simulink model "syntheses"  (R2015b)
settings: Solver=FixedStepDiscrete  SolverMode=SingleTasking  StartTime=0.0  StopTime=sim_len  FixedStep=1  RelTol=1e-3
values from neighbouring files (symbols this model uses):
  N_sub = 16    [synthese_params.m]
undefined symbols (not defined in the file or in its folder): modulator_reg_1_address, modulator_reg_1_default, modulator_reg_1_num_bits
undefined symbols (not defined in the file): reset_reg_address
libraries: xbsIndex_r4 x136
settings Model: Creator=randy  LastModifiedBy=randy

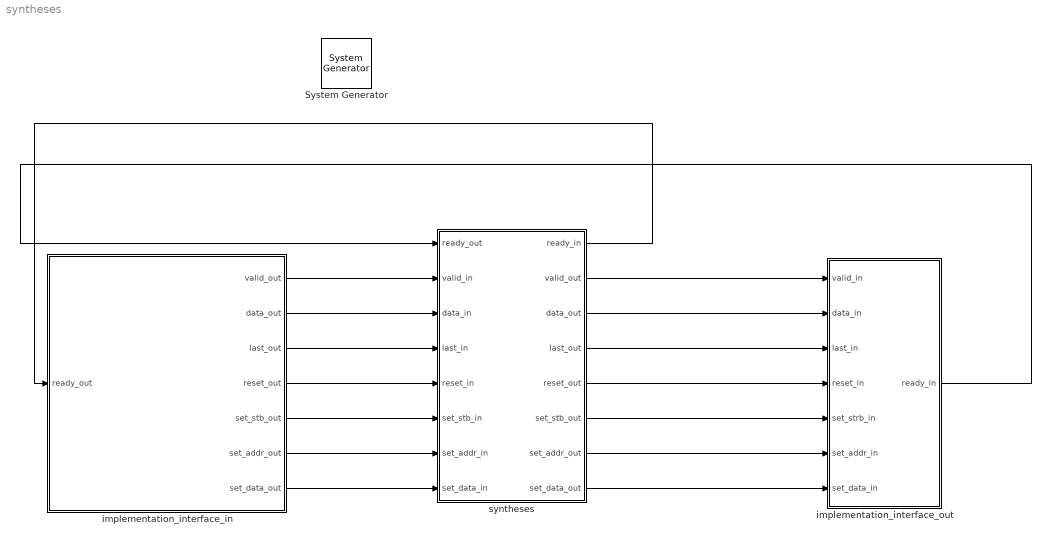
== system syntheses ==
  " System Generator" : xbsIndex_r4/ System Generator  Tag=genX  xilinxfamily=kintex7  part=xc7k410t  speed=-2  package=ffg900  synthesis_tool=Vivado  clock_wrapper=Clock Enables  directory=./checkpoint  proj_type=Vivado  Synth_file=Vivado Synthesis Defaults  Impl_file=Vivado Implementation Defaults  testbench=off  simulink_period=1  sysclk_period=5  dcm_input_clock_period=10  incr_netlist=off  trim_vbits=Everywhere in SubSystem  dbl_ovrd=According to Block Masks  core_generation=According to Block Masks  run_coregen=off  deprecated_control=off  eval_field=0  block_type=sysgen
  implementation_interface_in : Subsystem
  implementation_interface_out : Subsystem
  syntheses : Subsystem
  wires:
  implementation_interface_in/1(valid_out) -> syntheses/2(valid_in)
  implementation_interface_in/2(data_out) -> syntheses/3(data_in)
  implementation_interface_in/3(last_out) -> syntheses/4(last_in)
  syntheses/1(ready_in) -> implementation_interface_in/1(ready_out)
  syntheses/2(valid_out) -> implementation_interface_out/1(valid_in)
  syntheses/3(data_out) -> implementation_interface_out/2(data_in)
  syntheses/4(last_out) -> implementation_interface_out/3(last_in)
  implementation_interface_out/1(ready_in) -> syntheses/1(ready_out)
  implementation_interface_in/4(reset_out) -> syntheses/5(reset_in)
  implementation_interface_in/5(set_stb_out) -> syntheses/6(set_stb_in)
  implementation_interface_in/6(set_addr_out) -> syntheses/7(set_addr_in)
  implementation_interface_in/7(set_data_out) -> syntheses/8(set_data_in)
  syntheses/5(reset_out) -> implementation_interface_out/4(reset_in)
  syntheses/6(set_stb_out) -> implementation_interface_out/5(set_strb_in)
  syntheses/7(set_addr_out) -> implementation_interface_out/6(set_addr_in)
  syntheses/8(set_data_out) -> implementation_interface_out/7(set_data_in)

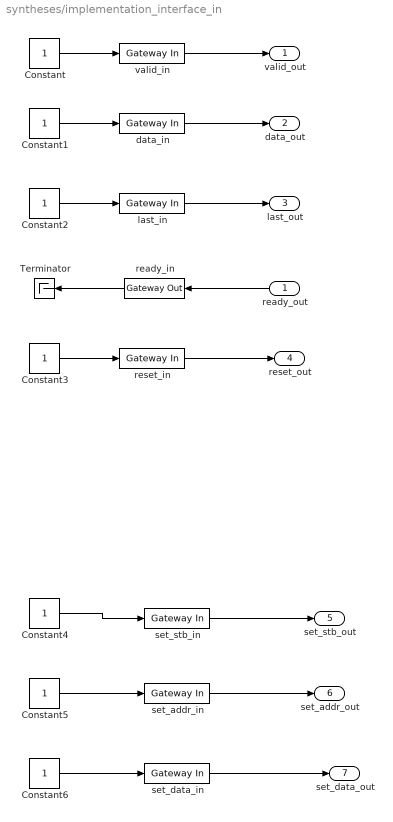
== system syntheses/implementation_interface_in ==
  ready_out : Inport
  Constant{,1..6} (7 alike) : Constant
  Terminator : Terminator
  data_in : xbsIndex_r4/Gateway In  gui_display_data_type=Fixed-point  arith_type=Unsigned  n_bits=32  bin_pt=0  preci_type=Single  exp_width=8  frac_width=24  rows=1  columns=1  quantization="Round  (unbiased: +/- Inf)"  overflow=Saturate  period=1  UseAsADC=off  ADCChannel='1'  interface=None  automatic_assignment=on  address_offset=hex2dec('00')  intf_name=''  intf_description=''  timing_constraint=None  locs_specified=off  LOCs={}  io_standard={}  inherit_from_input=off  hdl_port=on  dbl_ovrd=off  block_type=gatewayin
  last_in : xbsIndex_r4/Gateway In  gui_display_data_type=Boolean  arith_type=Boolean  n_bits=16  bin_pt=14  preci_type=Single  exp_width=8  frac_width=24  rows=1  columns=1  quantization="Round  (unbiased: +/- Inf)"  overflow=Saturate  period=1  UseAsADC=off  ADCChannel='1'  interface=None  automatic_assignment=on  address_offset=hex2dec('00')  intf_name=''  intf_description=''  timing_constraint=None  locs_specified=off  LOCs={}  io_standard={}  inherit_from_input=off  hdl_port=on  dbl_ovrd=off  block_type=gatewayin
  ready_in : xbsIndex_r4/Gateway Out  inherit_from_input=off  hdl_port=on  rows=1  columns=1  UseAsDAC=off  DACChannel='1'  interface=None  automatic_assignment=on  address_offset=hex2dec('00')  intf_name=''  intf_description=''  timing_constraint=None  locs_specified=off  LOCs={}  io_standard={}  block_type=gatewayout
  reset_in : xbsIndex_r4/Gateway In  gui_display_data_type=Boolean  arith_type=Boolean  n_bits=16  bin_pt=14  preci_type=Single  exp_width=8  frac_width=24  rows=1  columns=1  quantization="Round  (unbiased: +/- Inf)"  overflow=Saturate  period=1  UseAsADC=off  ADCChannel='1'  interface=None  automatic_assignment=on  address_offset=hex2dec('00')  intf_name=''  intf_description=''  timing_constraint=None  locs_specified=off  LOCs={}  io_standard={}  inherit_from_input=off  hdl_port=on  dbl_ovrd=off  block_type=gatewayin
  set_addr_in : xbsIndex_r4/Gateway In  gui_display_data_type=Fixed-point  arith_type=Unsigned  n_bits=8  bin_pt=0  preci_type=Single  exp_width=8  frac_width=24  rows=1  columns=1  quantization="Round  (unbiased: +/- Inf)"  overflow=Saturate  period=1  UseAsADC=off  ADCChannel='1'  interface=None  automatic_assignment=on  address_offset=hex2dec('00')  intf_name=''  intf_description=''  timing_constraint=None  locs_specified=off  LOCs={}  io_standard={}  inherit_from_input=off  hdl_port=on  dbl_ovrd=off  block_type=gatewayin
  set_data_in : xbsIndex_r4/Gateway In  gui_display_data_type=Fixed-point  arith_type=Unsigned  n_bits=32  bin_pt=0  preci_type=Single  exp_width=8  frac_width=24  rows=1  columns=1  quantization="Round  (unbiased: +/- Inf)"  overflow=Saturate  period=1  UseAsADC=off  ADCChannel='1'  interface=None  automatic_assignment=on  address_offset=hex2dec('00')  intf_name=''  intf_description=''  timing_constraint=None  locs_specified=off  LOCs={}  io_standard={}  inherit_from_input=off  hdl_port=on  dbl_ovrd=off  block_type=gatewayin
  set_stb_in : xbsIndex_r4/Gateway In  gui_display_data_type=Boolean  arith_type=Boolean  n_bits=16  bin_pt=14  preci_type=Single  exp_width=8  frac_width=24  rows=1  columns=1  quantization="Round  (unbiased: +/- Inf)"  overflow=Saturate  period=1  UseAsADC=off  ADCChannel='1'  interface=None  automatic_assignment=on  address_offset=hex2dec('00')  intf_name=''  intf_description=''  timing_constraint=None  locs_specified=off  LOCs={}  io_standard={}  inherit_from_input=off  hdl_port=on  dbl_ovrd=off  block_type=gatewayin
  valid_in : xbsIndex_r4/Gateway In  gui_display_data_type=Boolean  arith_type=Boolean  n_bits=16  bin_pt=14  preci_type=Single  exp_width=8  frac_width=24  rows=1  columns=1  quantization="Round  (unbiased: +/- Inf)"  overflow=Saturate  period=1  UseAsADC=off  ADCChannel='1'  interface=None  automatic_assignment=on  address_offset=hex2dec('00')  intf_name=''  intf_description=''  timing_constraint=None  locs_specified=off  LOCs={}  io_standard={}  inherit_from_input=off  hdl_port=on  dbl_ovrd=off  block_type=gatewayin
  valid_out : Outport
  data_out : Outport  Port=2
  last_out : Outport  Port=3
  reset_out : Outport  Port=4
  set_stb_out : Outport  Port=5
  set_addr_out : Outport  Port=6
  set_data_out : Outport  Port=7
  wires:
  set_stb_in/1 -> set_stb_out/1
  set_addr_in/1 -> set_addr_out/1
  set_data_in/1 -> set_data_out/1
  reset_in/1 -> reset_out/1
  ready_out/1 -> ready_in/1
  last_in/1 -> last_out/1
  data_in/1 -> data_out/1
  valid_in/1 -> valid_out/1
  ready_in/1 -> Terminator/1
  Constant/1 -> valid_in/1
  Constant1/1 -> data_in/1
  Constant3/1 -> reset_in/1
  Constant2/1 -> last_in/1
  Constant4/1 -> set_stb_in/1
  Constant5/1 -> set_addr_in/1
  Constant6/1 -> set_data_in/1

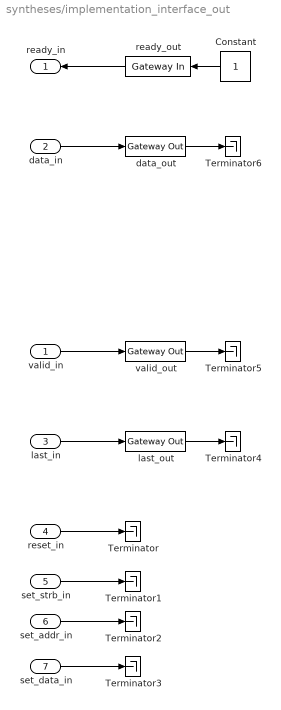
== system syntheses/implementation_interface_out ==
  valid_in : Inport
  data_in : Inport  Port=2
  last_in : Inport  Port=3
  reset_in : Inport  Port=4
  set_strb_in : Inport  Port=5
  set_addr_in : Inport  Port=6
  set_data_in : Inport  Port=7
  Constant : Constant
  Terminator{,1..6} (7 alike) : Terminator
  data_out : xbsIndex_r4/Gateway Out  inherit_from_input=off  hdl_port=on  rows=1  columns=1  UseAsDAC=off  DACChannel='1'  interface=None  automatic_assignment=on  address_offset=hex2dec('00')  intf_name=''  intf_description=''  timing_constraint=None  locs_specified=off  LOCs={}  io_standard={}  block_type=gatewayout
  last_out : xbsIndex_r4/Gateway Out  inherit_from_input=off  hdl_port=on  rows=1  columns=1  UseAsDAC=off  DACChannel='1'  interface=None  automatic_assignment=on  address_offset=hex2dec('00')  intf_name=''  intf_description=''  timing_constraint=None  locs_specified=off  LOCs={}  io_standard={}  block_type=gatewayout
  ready_out : xbsIndex_r4/Gateway In  gui_display_data_type=Boolean  arith_type=Boolean  n_bits=16  bin_pt=14  preci_type=Single  exp_width=8  frac_width=24  rows=1  columns=1  quantization="Round  (unbiased: +/- Inf)"  overflow=Saturate  period=1  UseAsADC=off  ADCChannel='1'  interface=None  automatic_assignment=on  address_offset=hex2dec('00')  intf_name=''  intf_description=''  timing_constraint=None  locs_specified=off  LOCs={}  io_standard={}  inherit_from_input=off  hdl_port=on  dbl_ovrd=off  block_type=gatewayin
  valid_out : xbsIndex_r4/Gateway Out  inherit_from_input=off  hdl_port=on  rows=1  columns=1  UseAsDAC=off  DACChannel='1'  interface=None  automatic_assignment=on  address_offset=hex2dec('00')  intf_name=''  intf_description=''  timing_constraint=None  locs_specified=off  LOCs={}  io_standard={}  block_type=gatewayout
  ready_in : Outport
  wires:
  valid_out/1 -> Terminator5/1
  Constant/1 -> ready_out/1
  last_out/1 -> Terminator4/1
  data_out/1 -> Terminator6/1
  reset_in/1 -> Terminator/1
  set_strb_in/1 -> Terminator1/1
  set_addr_in/1 -> Terminator2/1
  set_data_in/1 -> Terminator3/1
  valid_in/1 -> valid_out/1
  data_in/1 -> data_out/1
  last_in/1 -> last_out/1
  ready_out/1 -> ready_in/1

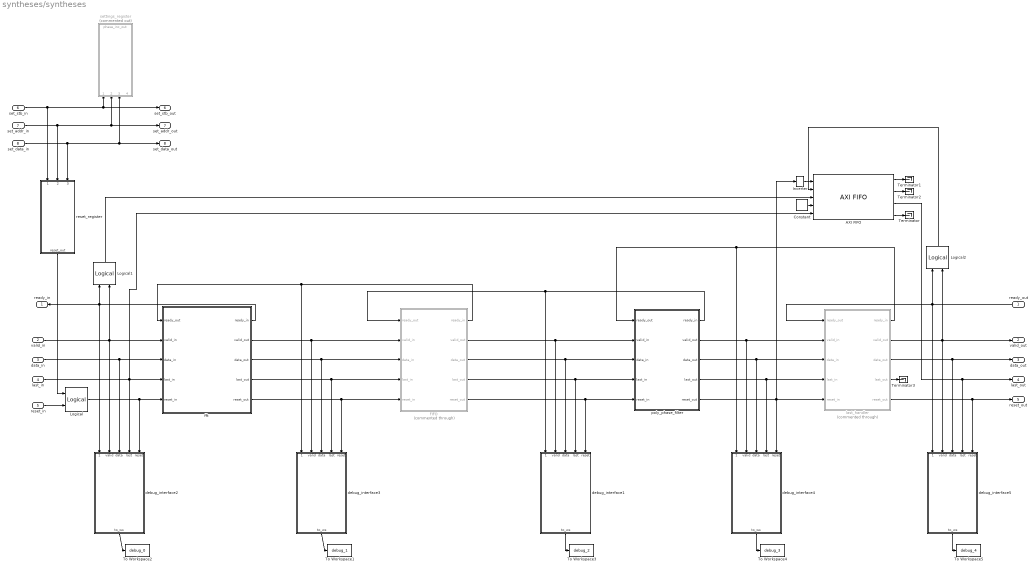
== system syntheses/syntheses ==
  ready_out : Inport
  valid_in : Inport  Port=2
  data_in : Inport  Port=3
  last_in : Inport  Port=4
  reset_in : Inport  Port=5
  set_stb_in : Inport  Port=6
  set_addr_in : Inport  Port=7
  set_data_in : Inport  Port=8
  AXI FIFO : xbsIndex_r4/AXI FIFO  input_depth_axis=4K  actual_fifo_depth_label=4098  enable_tdata=on  enable_tdest=off  enable_tstrb=off  enable_tready=on  enable_tid=off  enable_tuser=off  enable_tkeep=off  enable_tlast=on  has_aresetn=on  enable_data_counts_axis=off  fifo_implementation_type_axis=Common Clock Block RAM  trim_axipin_name=on  programmable_full_type_axis=Full  full_threshold_assert_value_axis=0  programmable_empty_type_axis=Empty  empty_threshold_assert_value_axis=1022  underflow_flag_axi=0  underflow_sense_axi=Active High  overflow_flag_axi=0  overflow_sense_axi=Active High  block_type=axi_fifo
  Constant : xbsIndex_r4/Constant  const=1.0  gui_display_data_type=Fixed-point  arith_type=Unsigned  n_bits=8  bin_pt=0  preci_type=Single  exp_width=8  frac_width=24  explicit_period=on  period=1  equ=P=C  opselect=C  inp2=PCIN>>17  opr=+  inp1=P  carry=CIN  dbl_ovrd=off  block_type=constant
  FIFO : Subsystem  Commented=through
  Inverter : xbsIndex_r4/Inverter  en=off  latency=0  dbl_ovrd=off  block_type=inv
  Logical : xbsIndex_r4/Logical  logical_function=OR  inputs=2  en=off  latency=0  precision=Full  arith_type=Unsigned  n_bits=16  bin_pt=0  align_bp=on  dbl_ovrd=off  block_type=logical
  Logical1 : xbsIndex_r4/Logical  logical_function=AND  inputs=2  en=off  latency=0  precision=Full  arith_type=Unsigned  n_bits=16  bin_pt=0  align_bp=on  dbl_ovrd=off  block_type=logical
  Logical2 : xbsIndex_r4/Logical  logical_function=AND  inputs=2  en=off  latency=0  precision=Full  arith_type=Unsigned  n_bits=16  bin_pt=0  align_bp=on  dbl_ovrd=off  block_type=logical
  Terminator{,1..3} (4 alike) : Terminator
  To Workspace1 : ToWorkspace  VariableName=debug_1  SaveFormat=Timeseries  SampleTime=-1
  To Workspace2 : ToWorkspace  VariableName=debug_0  SaveFormat=Timeseries  SampleTime=-1
  To Workspace3 : ToWorkspace  VariableName=debug_2  SaveFormat=Timeseries  SampleTime=-1
  To Workspace4 : ToWorkspace  VariableName=debug_3  SaveFormat=Timeseries  SampleTime=-1
  To Workspace5 : ToWorkspace  VariableName=debug_4  SaveFormat=Timeseries  SampleTime=-1
  debug_interface1 : Subsystem
  debug_interface2 : Subsystem
  debug_interface3 : Subsystem
  debug_interface4 : Subsystem
  debug_interface5 : Subsystem
  fft : Subsystem
  last_handler : Subsystem  Commented=through
  poly_phase_filter : Subsystem
  reset_register : Subsystem  mask{address=reset_reg_address}
  settings_register : Subsystem  Commented=on
  ready_in : Outport
  valid_out : Outport  Port=2
  data_out : Outport  Port=3
  last_out : Outport  Port=4
  reset_out : Outport  Port=5
  set_stb_out : Outport  Port=6
  set_addr_out : Outport  Port=7
  set_data_out : Outport  Port=8
  wires:
  set_addr_in/1 -> settings_register/2(set_addr), set_addr_out/1, reset_register/2(set_addr)
  set_data_in/1 -> settings_register/3(set_data), set_data_out/1, reset_register/3(set_data)
  debug_interface2/1(to_ws) -> To Workspace2/1
  debug_interface3/1(to_ws) -> To Workspace1/1
  debug_interface1/1(to_ws) -> To Workspace3/1
  debug_interface4/1(to_ws) -> To Workspace4/1
  fft/1(ready_in) -> Logical1/1, debug_interface2/1(ready), ready_in/1
  data_in/1 -> debug_interface2/3(data), fft/3(data_in)
  valid_in/1 -> Logical1/2, debug_interface2/2(valid), fft/2(valid_in)
  fft/2(valid_out) -> debug_interface3/2(valid), FIFO/2(valid_in)
  fft/3(data_out) -> debug_interface3/3(data), FIFO/3(data_in)
  fft/4(last_out) -> debug_interface3/4(last), FIFO/4(last_in)
  fft/5(reset_out) -> debug_interface3/5(reset), FIFO/5(reset_in)
  FIFO/2(valid_out) -> debug_interface1/2(valid), poly_phase_filter/2(valid_in)
  FIFO/3(data_out) -> debug_interface1/3(data), poly_phase_filter/3(data_in)
  FIFO/4(last_out) -> debug_interface1/4(last), poly_phase_filter/4(last_in)
  FIFO/5(reset_out) -> debug_interface1/5(reset), poly_phase_filter/5(reset_in)
  poly_phase_filter/1(ready_in) -> debug_interface1/1(ready), FIFO/1(ready_out)
  FIFO/1(ready_in) -> debug_interface3/1(ready), fft/1(ready_out)
  debug_interface5/1(to_ws) -> To Workspace5/1
  poly_phase_filter/2(valid_out) -> debug_interface4/2(valid), last_handler/2(valid_in)
  poly_phase_filter/3(data_out) -> last_handler/3(data_in), debug_interface4/3(data)
  poly_phase_filter/4(last_out) -> debug_interface4/4(last), last_handler/4(last_in)
  poly_phase_filter/5(reset_out) -> debug_interface4/5(reset), last_handler/5(reset_in), Inverter/1
  last_handler/1(ready_in) -> poly_phase_filter/1(ready_out), debug_interface4/1(ready)
  ready_out/1 -> Logical2/1, debug_interface5/1(ready), last_handler/1(ready_out)
  last_handler/2(valid_out) -> Logical2/2, debug_interface5/2(valid), valid_out/1
  last_handler/3(data_out) -> data_out/1, debug_interface5/3(data)
  last_handler/5(reset_out) -> reset_out/1, debug_interface5/5(reset)
  Logical/1 -> fft/5(reset_in), debug_interface2/5(reset)
  reset_in/1 -> Logical/2
  reset_register/1(reset_out) -> Logical/1
  set_stb_in/1 -> reset_register/1(set_stb), settings_register/1(set_stb), set_stb_out/1
  last_in/1 -> AXI FIFO/5, fft/4(last_in), debug_interface2/4(last)
  AXI FIFO/1 -> Terminator1/1
  Constant/1 -> AXI FIFO/4
  AXI FIFO/2 -> Terminator2/1
  AXI FIFO/4 -> Terminator/1
  Logical1/1 -> AXI FIFO/3
  Logical2/1 -> AXI FIFO/2
  AXI FIFO/3 -> last_out/1, debug_interface5/4(last)
  last_handler/4(last_out) -> Terminator3/1
  Inverter/1 -> AXI FIFO/1

== system syntheses/syntheses/FIFO ==
  ready_out : Inport
  valid_in : Inport  Port=2
  data_in : Inport  Port=3
  last_in : Inport  Port=4
  reset_in : Inport  Port=5
  AXI FIFO : xbsIndex_r4/AXI FIFO  input_depth_axis=16  actual_fifo_depth_label=18  enable_tdata=on  enable_tdest=off  enable_tstrb=off  enable_tready=on  enable_tid=off  enable_tuser=off  enable_tkeep=off  enable_tlast=on  has_aresetn=on  enable_data_counts_axis=off  fifo_implementation_type_axis=Common Clock Distributed RAM  trim_axipin_name=on  programmable_full_type_axis=Full  full_threshold_assert_value_axis=0  programmable_empty_type_axis=Empty  empty_threshold_assert_value_axis=1022  underflow_flag_axi=0  underflow_sense_axi=Active High  overflow_flag_axi=0  overflow_sense_axi=Active High  block_type=axi_fifo
  Inverter : xbsIndex_r4/Inverter  en=off  latency=0  dbl_ovrd=off  block_type=inv
  ready_in : Outport
  valid_out : Outport  Port=2
  data_out : Outport  Port=3
  last_out : Outport  Port=4
  reset_out : Outport  Port=5
  wires:
  AXI FIFO/1 -> valid_out/1
  data_in/1 -> AXI FIFO/4
  ready_out/1 -> AXI FIFO/2
  last_in/1 -> AXI FIFO/5
  AXI FIFO/3 -> last_out/1
  reset_in/1 -> reset_out/1, Inverter/1
  valid_in/1 -> AXI FIFO/3
  Inverter/1 -> AXI FIFO/1
  AXI FIFO/2 -> data_out/1
  AXI FIFO/4 -> ready_in/1

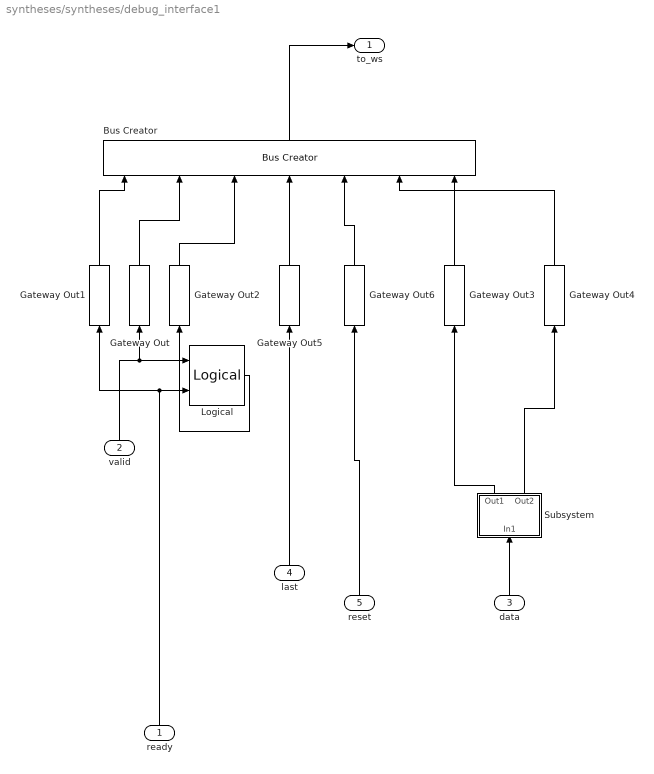
== system syntheses/syntheses/debug_interface1 ==
  ready : Inport
  valid : Inport  Port=2
  data : Inport  Port=3
  last : Inport  Port=4
  reset : Inport  Port=5
  Bus Creator : BusCreator  Inputs=7
  Gateway Out{,1..6} (7 alike) : xbsIndex_r4/Gateway Out  inherit_from_input=off  hdl_port=off  rows=1  columns=1  UseAsDAC=off  DACChannel='1'  interface=None  automatic_assignment=on  address_offset=hex2dec('00')  intf_name=''  intf_description=''  timing_constraint=None  locs_specified=off  LOCs={}  io_standard={}  block_type=gatewayout
  Logical : xbsIndex_r4/Logical  logical_function=AND  inputs=2  en=off  latency=0  precision=Full  arith_type=Unsigned  n_bits=16  bin_pt=0  align_bp=on  dbl_ovrd=off  block_type=logical
  Subsystem : Subsystem
  to_ws : Outport
  wires:
  ready/1 -> Logical/2, Gateway Out1/1
  Gateway Out3/1 -> Bus Creator/7
  Gateway Out2/1 -> Bus Creator/3
  Logical/1 -> Gateway Out2/1
  Gateway Out4/1 -> Bus Creator/6
  valid/1 -> Logical/1, Gateway Out/1
  Gateway Out1/1 -> Bus Creator/1
  Gateway Out/1 -> Bus Creator/2
  Gateway Out6/1 -> Bus Creator/5
  reset/1 -> Gateway Out6/1
  Bus Creator/1 -> to_ws/1
  Subsystem/1(Out1) -> Gateway Out3/1
  Subsystem/2(Out2) -> Gateway Out4/1
  data/1 -> Subsystem/1(In1)
  Gateway Out5/1 -> Bus Creator/4
  last/1 -> Gateway Out5/1

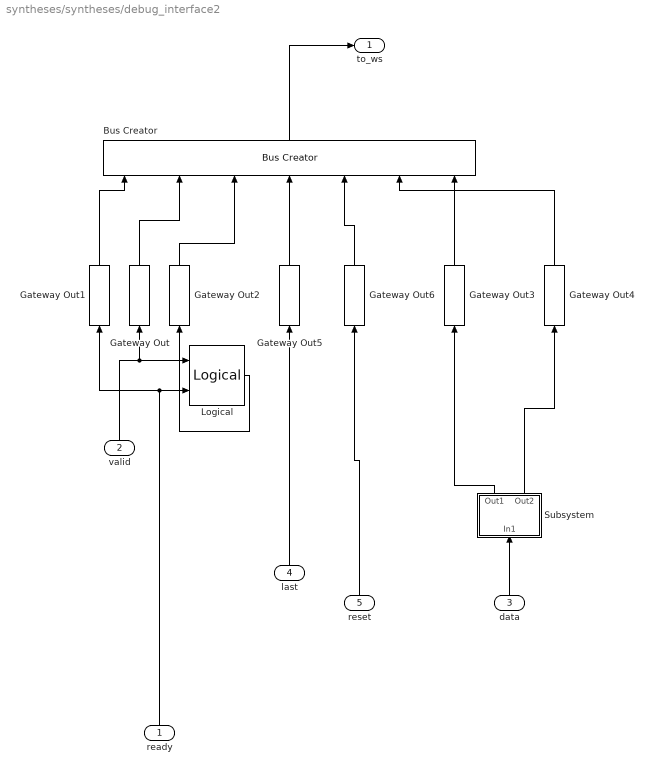
== system syntheses/syntheses/debug_interface2 ==
  ready : Inport
  valid : Inport  Port=2
  data : Inport  Port=3
  last : Inport  Port=4
  reset : Inport  Port=5
  Bus Creator : BusCreator  Inputs=7
  Gateway Out{,1..6} (7 alike) : xbsIndex_r4/Gateway Out  inherit_from_input=off  hdl_port=off  rows=1  columns=1  UseAsDAC=off  DACChannel='1'  interface=None  automatic_assignment=on  address_offset=hex2dec('00')  intf_name=''  intf_description=''  timing_constraint=None  locs_specified=off  LOCs={}  io_standard={}  block_type=gatewayout
  Logical : xbsIndex_r4/Logical  logical_function=AND  inputs=2  en=off  latency=0  precision=Full  arith_type=Unsigned  n_bits=16  bin_pt=0  align_bp=on  dbl_ovrd=off  block_type=logical
  Subsystem : Subsystem
  to_ws : Outport
  wires:
  ready/1 -> Logical/2, Gateway Out1/1
  Gateway Out3/1 -> Bus Creator/7
  Gateway Out2/1 -> Bus Creator/3
  Logical/1 -> Gateway Out2/1
  Gateway Out4/1 -> Bus Creator/6
  valid/1 -> Logical/1, Gateway Out/1
  Gateway Out1/1 -> Bus Creator/1
  Gateway Out/1 -> Bus Creator/2
  Gateway Out6/1 -> Bus Creator/5
  reset/1 -> Gateway Out6/1
  Bus Creator/1 -> to_ws/1
  Subsystem/1(Out1) -> Gateway Out3/1
  Subsystem/2(Out2) -> Gateway Out4/1
  data/1 -> Subsystem/1(In1)
  Gateway Out5/1 -> Bus Creator/4
  last/1 -> Gateway Out5/1

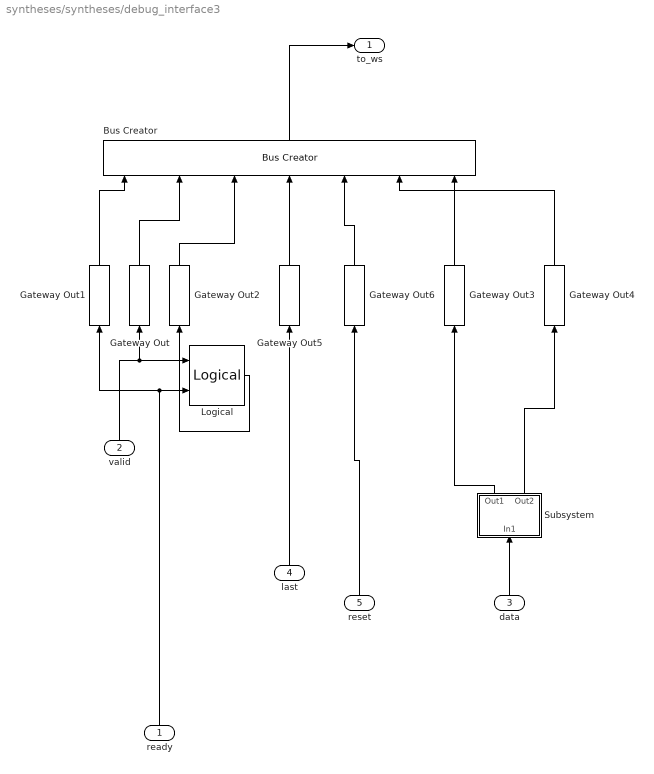
== system syntheses/syntheses/debug_interface3 ==
  ready : Inport
  valid : Inport  Port=2
  data : Inport  Port=3
  last : Inport  Port=4
  reset : Inport  Port=5
  Bus Creator : BusCreator  Inputs=7
  Gateway Out{,1..6} (7 alike) : xbsIndex_r4/Gateway Out  inherit_from_input=off  hdl_port=off  rows=1  columns=1  UseAsDAC=off  DACChannel='1'  interface=None  automatic_assignment=on  address_offset=hex2dec('00')  intf_name=''  intf_description=''  timing_constraint=None  locs_specified=off  LOCs={}  io_standard={}  block_type=gatewayout
  Logical : xbsIndex_r4/Logical  logical_function=AND  inputs=2  en=off  latency=0  precision=Full  arith_type=Unsigned  n_bits=16  bin_pt=0  align_bp=on  dbl_ovrd=off  block_type=logical
  Subsystem : Subsystem
  to_ws : Outport
  wires:
  last/1 -> Gateway Out5/1
  Gateway Out5/1 -> Bus Creator/4
  data/1 -> Subsystem/1(In1)
  Subsystem/2(Out2) -> Gateway Out4/1
  Subsystem/1(Out1) -> Gateway Out3/1
  Bus Creator/1 -> to_ws/1
  reset/1 -> Gateway Out6/1
  Gateway Out6/1 -> Bus Creator/5
  Gateway Out/1 -> Bus Creator/2
  Gateway Out1/1 -> Bus Creator/1
  valid/1 -> Gateway Out/1, Logical/1
  Gateway Out4/1 -> Bus Creator/6
  Logical/1 -> Gateway Out2/1
  Gateway Out2/1 -> Bus Creator/3
  Gateway Out3/1 -> Bus Creator/7
  ready/1 -> Gateway Out1/1, Logical/2

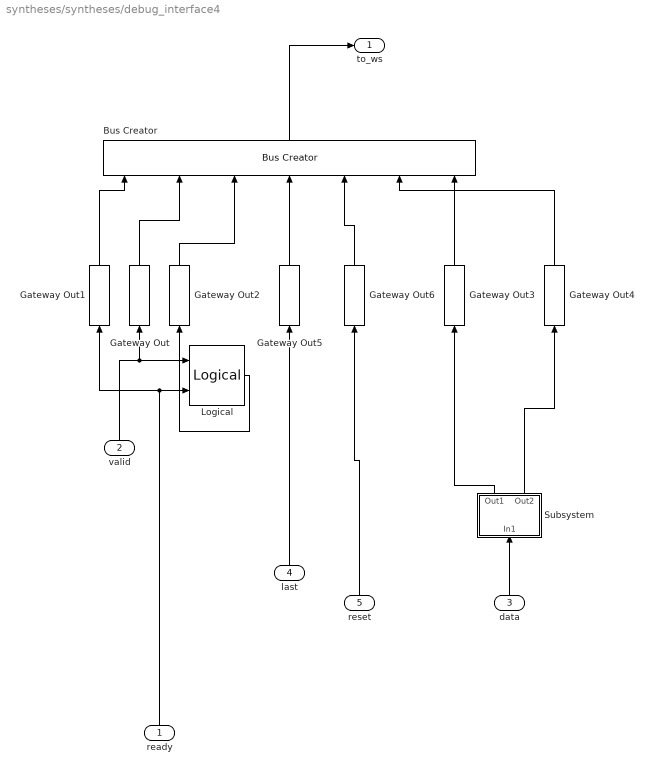
== system syntheses/syntheses/debug_interface4 ==
  ready : Inport
  valid : Inport  Port=2
  data : Inport  Port=3
  last : Inport  Port=4
  reset : Inport  Port=5
  Bus Creator : BusCreator  Inputs=7
  Gateway Out{,1..6} (7 alike) : xbsIndex_r4/Gateway Out  inherit_from_input=off  hdl_port=off  rows=1  columns=1  UseAsDAC=off  DACChannel='1'  interface=None  automatic_assignment=on  address_offset=hex2dec('00')  intf_name=''  intf_description=''  timing_constraint=None  locs_specified=off  LOCs={}  io_standard={}  block_type=gatewayout
  Logical : xbsIndex_r4/Logical  logical_function=AND  inputs=2  en=off  latency=0  precision=Full  arith_type=Unsigned  n_bits=16  bin_pt=0  align_bp=on  dbl_ovrd=off  block_type=logical
  Subsystem : Subsystem
  to_ws : Outport
  wires:
  ready/1 -> Logical/2, Gateway Out1/1
  Gateway Out3/1 -> Bus Creator/7
  Gateway Out2/1 -> Bus Creator/3
  Logical/1 -> Gateway Out2/1
  Gateway Out4/1 -> Bus Creator/6
  valid/1 -> Logical/1, Gateway Out/1
  Gateway Out1/1 -> Bus Creator/1
  Gateway Out/1 -> Bus Creator/2
  Gateway Out6/1 -> Bus Creator/5
  reset/1 -> Gateway Out6/1
  Bus Creator/1 -> to_ws/1
  Subsystem/1(Out1) -> Gateway Out3/1
  Subsystem/2(Out2) -> Gateway Out4/1
  data/1 -> Subsystem/1(In1)
  Gateway Out5/1 -> Bus Creator/4
  last/1 -> Gateway Out5/1

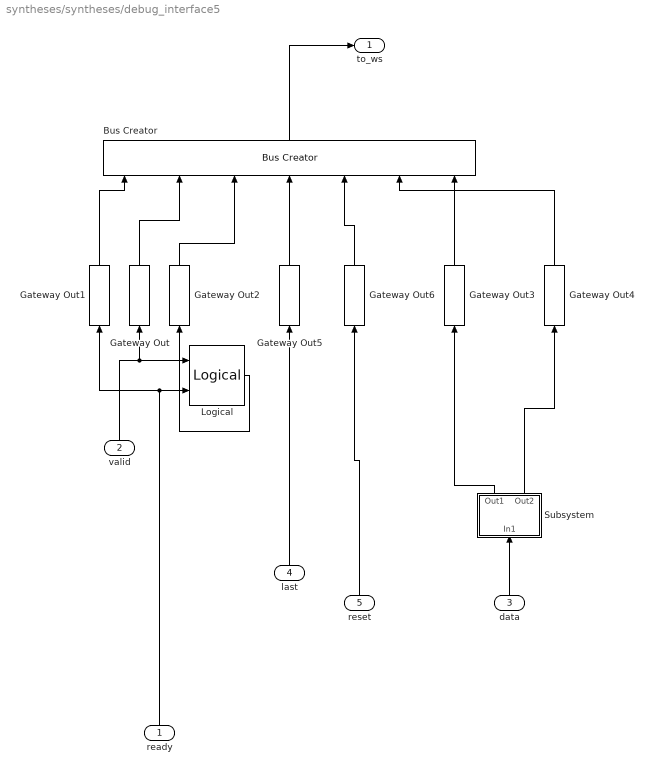
== system syntheses/syntheses/debug_interface5 ==
  ready : Inport
  valid : Inport  Port=2
  data : Inport  Port=3
  last : Inport  Port=4
  reset : Inport  Port=5
  Bus Creator : BusCreator  Inputs=7
  Gateway Out{,1..6} (7 alike) : xbsIndex_r4/Gateway Out  inherit_from_input=off  hdl_port=off  rows=1  columns=1  UseAsDAC=off  DACChannel='1'  interface=None  automatic_assignment=on  address_offset=hex2dec('00')  intf_name=''  intf_description=''  timing_constraint=None  locs_specified=off  LOCs={}  io_standard={}  block_type=gatewayout
  Logical : xbsIndex_r4/Logical  logical_function=AND  inputs=2  en=off  latency=0  precision=Full  arith_type=Unsigned  n_bits=16  bin_pt=0  align_bp=on  dbl_ovrd=off  block_type=logical
  Subsystem : Subsystem
  to_ws : Outport
  wires:
  ready/1 -> Logical/2, Gateway Out1/1
  Gateway Out3/1 -> Bus Creator/7
  Gateway Out2/1 -> Bus Creator/3
  Logical/1 -> Gateway Out2/1
  Gateway Out4/1 -> Bus Creator/6
  valid/1 -> Logical/1, Gateway Out/1
  Gateway Out1/1 -> Bus Creator/1
  Gateway Out/1 -> Bus Creator/2
  Gateway Out6/1 -> Bus Creator/5
  reset/1 -> Gateway Out6/1
  Bus Creator/1 -> to_ws/1
  Subsystem/1(Out1) -> Gateway Out3/1
  Subsystem/2(Out2) -> Gateway Out4/1
  data/1 -> Subsystem/1(In1)
  Gateway Out5/1 -> Bus Creator/4
  last/1 -> Gateway Out5/1

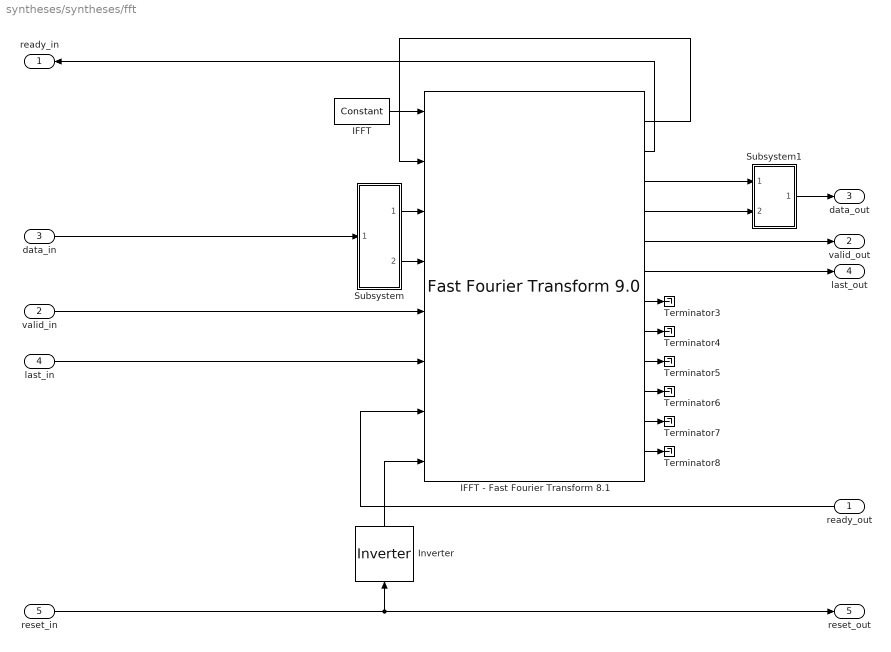
== system syntheses/syntheses/fft ==
  ready_out : Inport
  valid_in : Inport  Port=2
  data_in : Inport  Port=3
  last_in : Inport  Port=4
  reset_in : Inport  Port=5
  IFFT : xbsIndex_r4/Constant  const=0  gui_display_data_type=Fixed-point  arith_type=Unsigned  n_bits=1  bin_pt=0  preci_type=Single  exp_width=8  frac_width=24  explicit_period=off  period=1  equ=P=C  opselect=C  inp2=PCIN>>17  opr=+  inp1=P  carry=CIN  dbl_ovrd=off  block_type=constant
  IFFT - Fast Fourier Transform 8.1 : xbsIndex_r4/Fast Fourier Transform 9.0   transform_length=16  target_clock_frequency=200  target_data_throughput=50  implementation_options=pipelined_streaming_io  run_time_configurable_transform_length=off  phase_factor_width=17  scaling_options=unscaled  rounding_modes=convergent_rounding  aclken=off  aresetn=on  cyclic_prefix_insertion=off  output_ordering=natural_order  throttle_scheme=nonrealtime  xk_index=off  ovflo=off  trim_axipin_name=on  memory_options_data=block_ram  memory_options_phase_factors=block_ram  number_of_stages_using_block_ram_for_data_and_phase_factors=0  memory_options_reorder=block_ram  memory_options_hybrid=off  complex_mult_type=use_mults_resources  butterfly_type=use_xtremedsp_slices  simulation_type=hybrid_sim  simulation_model=sysgen:xfftv9_cmodel  data_path_portlist={ 's_axis_data_tdata', 'm_axis_data_tdata', 'm_axis_status_tdata', 'event_fft_overflow' }  channels=1  input_ordering=natural_order  input_width=16  ip_name=Fast Fourier Transform  ip_version=9.0  dsptool_ready=true  ipcore_usecache=true  ipcore_useipmodelcache=true  wrapper_available=true  port_translation_map={ 'aclken' => 'en', 'aresetn' => 'rst'}  data_format=fixed_point  block_type=xfft_v9_0
  Inverter : xbsIndex_r4/Inverter  en=off  latency=0  dbl_ovrd=off  block_type=inv
  Subsystem : Subsystem
  Subsystem1 : Subsystem
  Terminator{3..8} (6 alike) : Terminator
  ready_in : Outport
  valid_out : Outport  Port=2
  data_out : Outport  Port=3
  last_out : Outport  Port=4
  reset_out : Outport  Port=5
  wires:
  data_in/1 -> Subsystem/1(In1)
  IFFT - Fast Fourier Transform 8.1/10 -> Terminator6/1
  IFFT - Fast Fourier Transform 8.1/11 -> Terminator7/1
  IFFT - Fast Fourier Transform 8.1/8 -> Terminator4/1
  IFFT - Fast Fourier Transform 8.1/9 -> Terminator5/1
  IFFT - Fast Fourier Transform 8.1/7 -> Terminator3/1
  Subsystem/1(imag) -> IFFT - Fast Fourier Transform 8.1/3
  IFFT - Fast Fourier Transform 8.1/12 -> Terminator8/1
  Subsystem/2(real) -> IFFT - Fast Fourier Transform 8.1/4
  IFFT/1 -> IFFT - Fast Fourier Transform 8.1/1
  Subsystem1/1(Out1) -> data_out/1
  IFFT - Fast Fourier Transform 8.1/3 -> Subsystem1/1(imag)
  IFFT - Fast Fourier Transform 8.1/1 -> IFFT - Fast Fourier Transform 8.1/2
  IFFT - Fast Fourier Transform 8.1/4 -> Subsystem1/2(real)
  Inverter/1 -> IFFT - Fast Fourier Transform 8.1/8
  reset_in/1 -> Inverter/1, reset_out/1
  last_in/1 -> IFFT - Fast Fourier Transform 8.1/6
  valid_in/1 -> IFFT - Fast Fourier Transform 8.1/5
  IFFT - Fast Fourier Transform 8.1/2 -> ready_in/1
  IFFT - Fast Fourier Transform 8.1/5 -> valid_out/1
  ready_out/1 -> IFFT - Fast Fourier Transform 8.1/7
  IFFT - Fast Fourier Transform 8.1/6 -> last_out/1

== system syntheses/syntheses/last_handler ==
  ready_out : Inport
  valid_in : Inport  Port=2
  data_in : Inport  Port=3
  last_in : Inport  Port=4
  reset_in : Inport  Port=5
  Constant : xbsIndex_r4/Constant  const=1023  gui_display_data_type=Fixed-point  arith_type=Unsigned  n_bits=nextpow2(1024)  bin_pt=0  preci_type=Single  exp_width=8  frac_width=24  explicit_period=off  period=1  equ=P=C  opselect=C  inp2=PCIN>>17  opr=+  inp1=P  carry=CIN  dbl_ovrd=off  block_type=constant
  Counter : xbsIndex_r4/Counter  cnt_type=Free Running  cnt_to=Inf  operation=Up  start_count=0  cnt_by_val=1  arith_type=Unsigned  n_bits=nextpow2(1024)  bin_pt=0  load_pin=off  rst=on  en=on  explicit_period=on  period=1  use_behavioral_HDL=off  implementation=Fabric  dbl_ovrd=off  block_type=counter
  Logical : xbsIndex_r4/Logical  logical_function=AND  inputs=2  en=off  latency=0  precision=Full  arith_type=Unsigned  n_bits=16  bin_pt=0  align_bp=on  dbl_ovrd=off  block_type=logical
  Relational : xbsIndex_r4/Relational  mode=a=b  op_type=Bool  en=off  latency=0  dbl_ovrd=off  block_type=relational
  Terminator : Terminator
  ready_in : Outport
  valid_out : Outport  Port=2
  data_out : Outport  Port=3
  last_out : Outport  Port=4
  reset_out : Outport  Port=5
  wires:
  reset_in/1 -> Counter/1, reset_out/1
  ready_out/1 -> Logical/2, ready_in/1
  data_in/1 -> data_out/1
  valid_in/1 -> Logical/1, valid_out/1
  last_in/1 -> Terminator/1
  Logical/1 -> Counter/2
  Counter/1 -> Relational/2
  Constant/1 -> Relational/1
  Relational/1 -> last_out/1

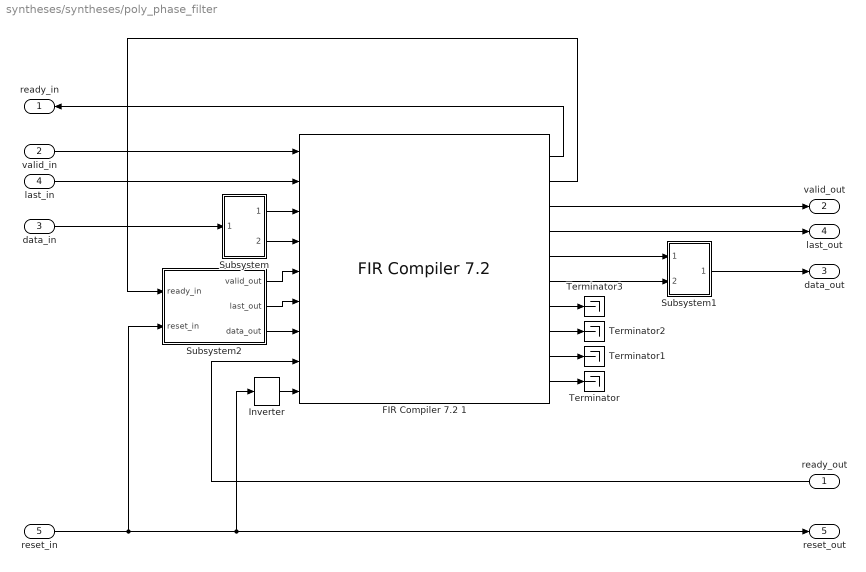
== system syntheses/syntheses/poly_phase_filter ==
  ready_out : Inport
  valid_in : Inport  Port=2
  data_in : Inport  Port=3
  last_in : Inport  Port=4
  reset_in : Inport  Port=5
  FIR Compiler 7.2 1 : xbsIndex_r4/FIR Compiler 7.2   coefficientvector=filt  coefficient_sets=N_sub  coefficient_reload=off  filter_type=Single_Rate  rate_change_type=Integer  interpolation_rate=1  decimation_rate=1  zero_pack_factor=1  channel_sequence=Basic  number_channels=N_sub  pattern_list='P4-0,P4-1,P4-2,P4-3,P4-4'  number_paths=2  ratespecification=Input_Sample_Period  sampleperiod=1  hardwareoversamplingrate=1  coefficient_sign=Signed  quantization=Quantize_Only  coefficient_width=16  bestprecision=off  coefficient_fractional_bits=14  coefficient_structure=Inferred  output_rounding_mode=Full_Precision  output_width=32  filter_architecture=Systolic_Multiply_Accumulate  optimization_goal=Area  optimization_list='None'  data_buffer_type=Automatic  coefficient_buffer_type=Automatic  input_buffer_type=Automatic  output_buffer_type=Automatic  preference_for_other_storage=Automatic  multi_column_support=Automatic  columnconfig='89'  inter_column_pipe_length=4  data_has_tlast=Vector_Framing  m_data_has_tready=on  s_data_has_fifo=on  s_data_has_tuser=Not_Required  m_data_has_tuser=Not_Required  s_config_sync_mode=On_Vector  s_config_method=By_Channel  num_reload_slots=1  has_aclken=off  has_aresetn=on  infoeditControl=ARESETn must be asserted for a minimum of 2 cycles  reset_data_vector=on  trim_axipin_name=on  simulation_type=hybrid_sim  simulation_model=sysgen:xfirv7_2_cmodel  data_path_portlist={ 's_axis_data_tdata', 'm_axis_data_tdata' }  passband_min=0.0  passband_max=0.5  stopband_min=0.5  stopband_max=1.0  filter_selection=1  gui_behaviour='Sysgen_GUI'  data_sign=Signed  data_width=16  data_fractional_bits=0  data_tuser_width=1  wrapper_available=true  ip_wrap_arbitrary_binary_point=true  ip_name=FIR Compiler  ip_version=7.2  dsptool_ready=true  ipcore_usecache=true  ipcore_useipmodelcache=true  port_translation_map={ 'aclken' => 'en', 'aresetn' => 'rst' }  run_core_at_system_period=true  ipcore_xco_need_fpga_part=true  block_type=fir_compiler_v7_2
      settings: infoedit=Maximum Possible : Maximizes oversampling rate. Abstracted input handshake (no s_data_tvalid) and automatic rate propagation.<br>Hardware Oversampling Rate : Specifies oversampling rate relative to the input sample period. Abstracted input handshake (no s_data_tvalid) and automatic rate propagation.<br>Input/Output Sample Period : Specifies absolute oversampling rate. No input handshake abstraction (exposes s_data_tvalid) and no rate propagation.
  Inverter : xbsIndex_r4/Inverter  en=off  latency=0  dbl_ovrd=off  block_type=inv
  Subsystem : Subsystem
  Subsystem1 : Subsystem
  Subsystem2 : Subsystem
  Terminator{,1..3} (4 alike) : Terminator
  ready_in : Outport
  valid_out : Outport  Port=2
  data_out : Outport  Port=3
  last_out : Outport  Port=4
  reset_out : Outport  Port=5
  wires:
  Subsystem1/1(Out1) -> data_out/1
  data_in/1 -> Subsystem/1(In1)
  valid_in/1 -> FIR Compiler 7.2 1/1
  last_in/1 -> FIR Compiler 7.2 1/2
  FIR Compiler 7.2 1/1 -> ready_in/1
  FIR Compiler 7.2 1/5 -> Subsystem1/1(imag)
  FIR Compiler 7.2 1/6 -> Subsystem1/2(real)
  ready_out/1 -> FIR Compiler 7.2 1/8
  reset_in/1 -> Subsystem2/2(reset_in), Inverter/1, reset_out/1
  Subsystem/1(imag) -> FIR Compiler 7.2 1/3
  Subsystem/2(real) -> FIR Compiler 7.2 1/4
  Inverter/1 -> FIR Compiler 7.2 1/9
  FIR Compiler 7.2 1/10 -> Terminator/1
  FIR Compiler 7.2 1/9 -> Terminator1/1
  FIR Compiler 7.2 1/8 -> Terminator2/1
  FIR Compiler 7.2 1/7 -> Terminator3/1
  FIR Compiler 7.2 1/3 -> valid_out/1
  FIR Compiler 7.2 1/4 -> last_out/1
  FIR Compiler 7.2 1/2 -> Subsystem2/1(ready_in)
  Subsystem2/3(data_out) -> FIR Compiler 7.2 1/7
  Subsystem2/2(last_out) -> FIR Compiler 7.2 1/6
  Subsystem2/1(valid_out) -> FIR Compiler 7.2 1/5

== system syntheses/syntheses/reset_register ==
  set_stb : Inport
  set_addr : Inport  Port=2
  set_data : Inport  Port=3
  Constant : xbsIndex_r4/Constant  const=1.0  gui_display_data_type=Boolean  arith_type=Boolean  n_bits=16  bin_pt=14  preci_type=Single  exp_width=8  frac_width=24  explicit_period=off  period=1  equ=P=C  opselect=C  inp2=PCIN>>17  opr=+  inp1=P  carry=CIN  dbl_ovrd=off  block_type=constant
  Counter : xbsIndex_r4/Counter  cnt_type=Free Running  cnt_to=Inf  operation=Up  start_count=0  cnt_by_val=1  arith_type=Unsigned  n_bits=2  bin_pt=0  load_pin=off  rst=on  en=on  explicit_period=on  period=1  use_behavioral_HDL=off  implementation=Fabric  dbl_ovrd=off  block_type=counter
  Delay : xbsIndex_r4/Delay  rst=on  infoeditControl=Selection of Reset will increase slice count due to use of real FFs and instead of SRLs  en=on  latency=1  reg_retiming=off  dbl_ovrd=off  block_type=delay
  Logical : xbsIndex_r4/Logical  logical_function=AND  inputs=2  en=off  latency=0  precision=Full  arith_type=Unsigned  n_bits=16  bin_pt=0  align_bp=on  dbl_ovrd=off  block_type=logical
  Relational : xbsIndex_r4/Relational  mode=a=b  op_type=Bool  en=off  latency=0  dbl_ovrd=off  block_type=relational
  Relational1 : xbsIndex_r4/Relational  mode=a=b  op_type=Bool  en=off  latency=0  dbl_ovrd=off  block_type=relational
  Terminator1 : Terminator
  address : xbsIndex_r4/Constant  const=address  gui_display_data_type=Fixed-point  arith_type=Unsigned  n_bits=8  bin_pt=0  preci_type=Single  exp_width=8  frac_width=24  explicit_period=off  period=1  equ=P=C  opselect=C  inp2=PCIN>>17  opr=+  inp1=P  carry=CIN  dbl_ovrd=off  block_type=constant
  address1 : xbsIndex_r4/Constant  const=3  gui_display_data_type=Fixed-point  arith_type=Unsigned  n_bits=2  bin_pt=0  preci_type=Single  exp_width=8  frac_width=24  explicit_period=off  period=1  equ=P=C  opselect=C  inp2=PCIN>>17  opr=+  inp1=P  carry=CIN  dbl_ovrd=off  block_type=constant
  reset_out : Outport
  wires:
  Relational/1 -> Logical/2
  address/1 -> Relational/2
  set_addr/1 -> Relational/1
  set_data/1 -> Terminator1/1
  Logical/1 -> Delay/3
  Constant/1 -> Delay/1
  Delay/1 -> reset_out/1, Counter/2
  Counter/1 -> Relational1/1
  address1/1 -> Relational1/2
  Relational1/1 -> Counter/1, Delay/2
  set_stb/1 -> Logical/1

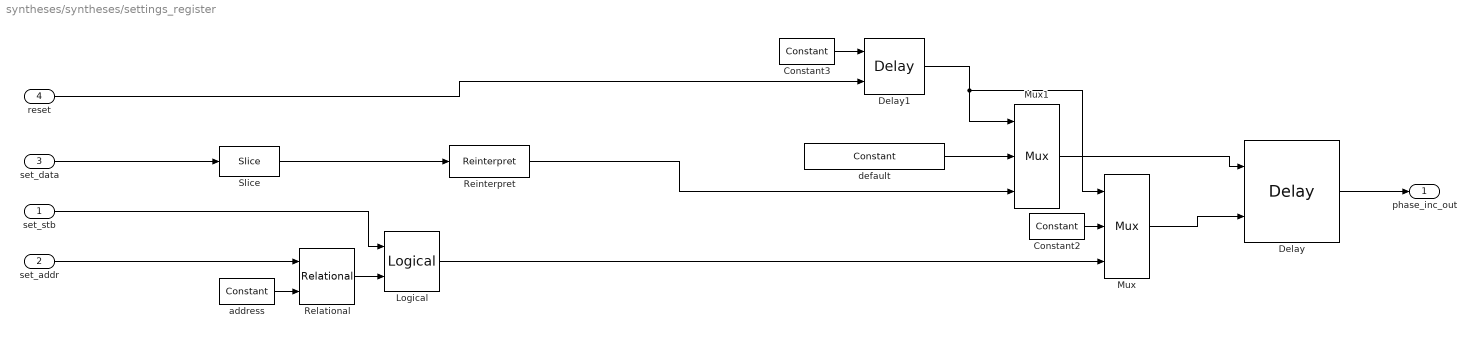
== system syntheses/syntheses/settings_register ==
  set_stb : Inport
  set_addr : Inport  Port=2
  set_data : Inport  Port=3
  reset : Inport  Port=4
  Constant2 : xbsIndex_r4/Constant  const=1.0  gui_display_data_type=Boolean  arith_type=Boolean  n_bits=16  bin_pt=14  preci_type=Single  exp_width=8  frac_width=24  explicit_period=off  period=1  equ=P=C  opselect=C  inp2=PCIN>>17  opr=+  inp1=P  carry=CIN  dbl_ovrd=off  block_type=constant
  Constant3 : xbsIndex_r4/Constant  const=1  gui_display_data_type=Boolean  arith_type=Boolean  n_bits=16  bin_pt=14  preci_type=Single  exp_width=8  frac_width=24  explicit_period=off  period=1  equ=P=C  opselect=C  inp2=PCIN>>17  opr=+  inp1=P  carry=CIN  dbl_ovrd=off  block_type=constant
  Delay : xbsIndex_r4/Delay  rst=off  infoeditControl=Selection of Reset will increase slice count due to use of real FFs and instead of SRLs  en=on  latency=1  reg_retiming=off  dbl_ovrd=off  block_type=delay
  Delay1 : xbsIndex_r4/Delay  rst=on  infoeditControl=Selection of Reset will increase slice count due to use of real FFs and instead of SRLs  en=off  latency=1  reg_retiming=off  dbl_ovrd=off  block_type=delay
  Logical : xbsIndex_r4/Logical  logical_function=AND  inputs=2  en=off  latency=0  precision=Full  arith_type=Unsigned  n_bits=16  bin_pt=0  align_bp=on  dbl_ovrd=off  block_type=logical
  Mux : xbsIndex_r4/Mux  inputs=2  en=off  latency=0  precision=Full  arith_type=Unsigned  n_bits=16  bin_pt=14  quantization=Truncate  overflow=Wrap  dbl_ovrd=off  block_type=mux
  Mux1 : xbsIndex_r4/Mux  inputs=2  en=off  latency=0  precision=Full  arith_type=Unsigned  n_bits=16  bin_pt=14  quantization=Truncate  overflow=Wrap  dbl_ovrd=off  block_type=mux
  Reinterpret : xbsIndex_r4/Reinterpret  force_arith_type=on  arith_type="Signed  (2's comp)"  force_bin_pt=on  bin_pt=modulator_reg_1_num_frac_bits  block_type=reinterpret
  Relational : xbsIndex_r4/Relational  mode=a=b  op_type=Bool  en=off  latency=0  dbl_ovrd=off  block_type=relational
  Slice : xbsIndex_r4/Slice  nbits=1  boolean_output=off  mode=Two Bit Locations  bit1=modulator_reg_1_num_bits-1  base1=LSB of Input  bit0=0  base0=LSB of Input  dbl_ovrd=off  block_type=slice
  address : xbsIndex_r4/Constant  const=modulator_reg_1_address  gui_display_data_type=Fixed-point  arith_type=Unsigned  n_bits=8  bin_pt=0  preci_type=Single  exp_width=8  frac_width=24  explicit_period=off  period=1  equ=P=C  opselect=C  inp2=PCIN>>17  opr=+  inp1=P  carry=CIN  dbl_ovrd=off  block_type=constant
  default : xbsIndex_r4/Constant  const=modulator_reg_1_default  gui_display_data_type=Fixed-point  arith_type=Signed (2's comp)  n_bits=modulator_reg_1_num_bits  bin_pt=modulator_reg_1_num_frac_bits  preci_type=Single  exp_width=8  frac_width=24  explicit_period=off  period=1  equ=P=C  opselect=C  inp2=PCIN>>17  opr=+  inp1=P  carry=CIN  dbl_ovrd=off  block_type=constant
  phase_inc_out : Outport
  wires:
  Relational/1 -> Logical/2
  address/1 -> Relational/2
  Delay/1 -> phase_inc_out/1
  set_data/1 -> Slice/1
  set_stb/1 -> Logical/1
  set_addr/1 -> Relational/1
  Slice/1 -> Reinterpret/1
  Constant3/1 -> Delay1/1
  Delay1/1 -> Mux/1, Mux1/1
  Mux/1 -> Delay/2
  Mux1/1 -> Delay/1
  Constant2/1 -> Mux/2
  default/1 -> Mux1/2
  Logical/1 -> Mux/3
  Reinterpret/1 -> Mux1/3
  reset/1 -> Delay1/2

== system syntheses/syntheses/debug_interface1/Subsystem ==
  In1 : Inport
  Reinterpret : xbsIndex_r4/Reinterpret  force_arith_type=on  arith_type="Signed  (2's comp)"  force_bin_pt=on  bin_pt=15  block_type=reinterpret
  Reinterpret3 : xbsIndex_r4/Reinterpret  force_arith_type=on  arith_type="Signed  (2's comp)"  force_bin_pt=on  bin_pt=15  block_type=reinterpret
  lower : xbsIndex_r4/Slice  nbits=1  boolean_output=off  mode=Two Bit Locations  bit1=15  base1=LSB of Input  bit0=0  base0=LSB of Input  dbl_ovrd=off  block_type=slice
  upper : xbsIndex_r4/Slice  nbits=1  boolean_output=off  mode=Two Bit Locations  bit1=31  base1=LSB of Input  bit0=16  base0=LSB of Input  dbl_ovrd=off  block_type=slice
  Out1 : Outport
  Out2 : Outport  Port=2
  wires:
  lower/1 -> Reinterpret/1
  In1/1 -> lower/1, upper/1
  upper/1 -> Reinterpret3/1
  Reinterpret3/1 -> Out1/1
  Reinterpret/1 -> Out2/1

== system syntheses/syntheses/debug_interface2/Subsystem ==
  In1 : Inport
  Reinterpret : xbsIndex_r4/Reinterpret  force_arith_type=on  arith_type="Signed  (2's comp)"  force_bin_pt=on  bin_pt=15  block_type=reinterpret
  Reinterpret3 : xbsIndex_r4/Reinterpret  force_arith_type=on  arith_type="Signed  (2's comp)"  force_bin_pt=on  bin_pt=15  block_type=reinterpret
  lower : xbsIndex_r4/Slice  nbits=1  boolean_output=off  mode=Two Bit Locations  bit1=15  base1=LSB of Input  bit0=0  base0=LSB of Input  dbl_ovrd=off  block_type=slice
  upper : xbsIndex_r4/Slice  nbits=1  boolean_output=off  mode=Two Bit Locations  bit1=31  base1=LSB of Input  bit0=16  base0=LSB of Input  dbl_ovrd=off  block_type=slice
  Out1 : Outport
  Out2 : Outport  Port=2
  wires:
  lower/1 -> Reinterpret/1
  In1/1 -> lower/1, upper/1
  upper/1 -> Reinterpret3/1
  Reinterpret3/1 -> Out1/1
  Reinterpret/1 -> Out2/1

== system syntheses/syntheses/debug_interface3/Subsystem ==
  In1 : Inport
  Reinterpret : xbsIndex_r4/Reinterpret  force_arith_type=on  arith_type="Signed  (2's comp)"  force_bin_pt=on  bin_pt=15  block_type=reinterpret
  Reinterpret3 : xbsIndex_r4/Reinterpret  force_arith_type=on  arith_type="Signed  (2's comp)"  force_bin_pt=on  bin_pt=15  block_type=reinterpret
  lower : xbsIndex_r4/Slice  nbits=1  boolean_output=off  mode=Two Bit Locations  bit1=15  base1=LSB of Input  bit0=0  base0=LSB of Input  dbl_ovrd=off  block_type=slice
  upper : xbsIndex_r4/Slice  nbits=1  boolean_output=off  mode=Two Bit Locations  bit1=31  base1=LSB of Input  bit0=16  base0=LSB of Input  dbl_ovrd=off  block_type=slice
  Out1 : Outport
  Out2 : Outport  Port=2
  wires:
  Reinterpret/1 -> Out2/1
  Reinterpret3/1 -> Out1/1
  upper/1 -> Reinterpret3/1
  In1/1 -> upper/1, lower/1
  lower/1 -> Reinterpret/1

== system syntheses/syntheses/debug_interface4/Subsystem ==
  In1 : Inport
  Reinterpret : xbsIndex_r4/Reinterpret  force_arith_type=on  arith_type="Signed  (2's comp)"  force_bin_pt=on  bin_pt=15  block_type=reinterpret
  Reinterpret3 : xbsIndex_r4/Reinterpret  force_arith_type=on  arith_type="Signed  (2's comp)"  force_bin_pt=on  bin_pt=15  block_type=reinterpret
  lower : xbsIndex_r4/Slice  nbits=1  boolean_output=off  mode=Two Bit Locations  bit1=15  base1=LSB of Input  bit0=0  base0=LSB of Input  dbl_ovrd=off  block_type=slice
  upper : xbsIndex_r4/Slice  nbits=1  boolean_output=off  mode=Two Bit Locations  bit1=31  base1=LSB of Input  bit0=16  base0=LSB of Input  dbl_ovrd=off  block_type=slice
  Out1 : Outport
  Out2 : Outport  Port=2
  wires:
  lower/1 -> Reinterpret/1
  In1/1 -> lower/1, upper/1
  upper/1 -> Reinterpret3/1
  Reinterpret3/1 -> Out1/1
  Reinterpret/1 -> Out2/1

== system syntheses/syntheses/debug_interface5/Subsystem ==
  In1 : Inport
  Reinterpret : xbsIndex_r4/Reinterpret  force_arith_type=on  arith_type="Signed  (2's comp)"  force_bin_pt=on  bin_pt=15  block_type=reinterpret
  Reinterpret3 : xbsIndex_r4/Reinterpret  force_arith_type=on  arith_type="Signed  (2's comp)"  force_bin_pt=on  bin_pt=15  block_type=reinterpret
  lower : xbsIndex_r4/Slice  nbits=1  boolean_output=off  mode=Two Bit Locations  bit1=15  base1=LSB of Input  bit0=0  base0=LSB of Input  dbl_ovrd=off  block_type=slice
  upper : xbsIndex_r4/Slice  nbits=1  boolean_output=off  mode=Two Bit Locations  bit1=31  base1=LSB of Input  bit0=16  base0=LSB of Input  dbl_ovrd=off  block_type=slice
  Out1 : Outport
  Out2 : Outport  Port=2
  wires:
  lower/1 -> Reinterpret/1
  In1/1 -> lower/1, upper/1
  upper/1 -> Reinterpret3/1
  Reinterpret3/1 -> Out1/1
  Reinterpret/1 -> Out2/1

== system syntheses/syntheses/fft/Subsystem ==
  In1 : Inport
  Reinterpret : xbsIndex_r4/Reinterpret  force_arith_type=on  arith_type="Signed  (2's comp)"  force_bin_pt=on  bin_pt=15  block_type=reinterpret
  Reinterpret1 : xbsIndex_r4/Reinterpret  force_arith_type=on  arith_type="Signed  (2's comp)"  force_bin_pt=on  bin_pt=15  block_type=reinterpret
  Slice : xbsIndex_r4/Slice  nbits=1  boolean_output=off  mode=Two Bit Locations  bit1=15  base1=LSB of Input  bit0=0  base0=LSB of Input  dbl_ovrd=off  block_type=slice
  Slice1 : xbsIndex_r4/Slice  nbits=1  boolean_output=off  mode=Two Bit Locations  bit1=31  base1=LSB of Input  bit0=16  base0=LSB of Input  dbl_ovrd=off  block_type=slice
  imag : Outport
  real : Outport  Port=2
  wires:
  Reinterpret1/1 -> imag/1
  In1/1 -> Slice1/1, Slice/1
  Reinterpret/1 -> real/1
  Slice1/1 -> Reinterpret1/1
  Slice/1 -> Reinterpret/1

== system syntheses/syntheses/fft/Subsystem1 ==
  imag : Inport
  real : Inport  Port=2
  Concat : xbsIndex_r4/Concat  num_inputs=2  dbl_ovrd=off  block_type=concat
  Convert : xbsIndex_r4/Convert  gui_display_data_type=Fixed-point  arith_type="Signed  (2's comp)"  n_bits=16  bin_pt=13  float_type=Single  exp_bits=8  fraction_bits=24  quantization=Truncate  overflow=Saturate  en=off  latency=0  pipeline=off  dbl_ovrd=off  block_type=convert
  Convert2 : xbsIndex_r4/Convert  gui_display_data_type=Fixed-point  arith_type="Signed  (2's comp)"  n_bits=16  bin_pt=13  float_type=Single  exp_bits=8  fraction_bits=24  quantization=Truncate  overflow=Saturate  en=off  latency=0  pipeline=off  dbl_ovrd=off  block_type=convert
  Reinterpret1 : xbsIndex_r4/Reinterpret  force_arith_type=on  arith_type=Unsigned  force_bin_pt=on  bin_pt=0  block_type=reinterpret
  Reinterpret2 : xbsIndex_r4/Reinterpret  force_arith_type=on  arith_type=Unsigned  force_bin_pt=on  bin_pt=0  block_type=reinterpret
  Out1 : Outport
  wires:
  Reinterpret1/1 -> Concat/2
  imag/1 -> Convert/1
  Concat/1 -> Out1/1
  Reinterpret2/1 -> Concat/1
  real/1 -> Convert2/1
  Convert/1 -> Reinterpret2/1
  Convert2/1 -> Reinterpret1/1

== system syntheses/syntheses/poly_phase_filter/Subsystem ==
  In1 : Inport
  Convert : xbsIndex_r4/Convert  gui_display_data_type=Fixed-point  arith_type="Signed  (2's comp)"  n_bits=18  bin_pt=0  float_type=Single  exp_bits=8  fraction_bits=24  quantization=Truncate  overflow=Wrap  en=off  latency=0  pipeline=off  dbl_ovrd=off  block_type=convert
  Convert1 : xbsIndex_r4/Convert  gui_display_data_type=Fixed-point  arith_type="Signed  (2's comp)"  n_bits=18  bin_pt=0  float_type=Single  exp_bits=8  fraction_bits=24  quantization=Truncate  overflow=Wrap  en=off  latency=0  pipeline=off  dbl_ovrd=off  block_type=convert
  Reinterpret : xbsIndex_r4/Reinterpret  force_arith_type=on  arith_type="Signed  (2's comp)"  force_bin_pt=on  bin_pt=0  block_type=reinterpret
  Reinterpret3 : xbsIndex_r4/Reinterpret  force_arith_type=on  arith_type="Signed  (2's comp)"  force_bin_pt=on  bin_pt=0  block_type=reinterpret
  lower : xbsIndex_r4/Slice  nbits=1  boolean_output=off  mode=Two Bit Locations  bit1=15  base1=LSB of Input  bit0=0  base0=LSB of Input  dbl_ovrd=off  block_type=slice
  upper : xbsIndex_r4/Slice  nbits=1  boolean_output=off  mode=Two Bit Locations  bit1=31  base1=LSB of Input  bit0=16  base0=LSB of Input  dbl_ovrd=off  block_type=slice
  imag : Outport
  real : Outport  Port=2
  wires:
  lower/1 -> Reinterpret/1
  Reinterpret/1 -> Convert1/1
  In1/1 -> lower/1, upper/1
  upper/1 -> Reinterpret3/1
  Reinterpret3/1 -> Convert/1
  Convert/1 -> imag/1
  Convert1/1 -> real/1

== system syntheses/syntheses/poly_phase_filter/Subsystem1 ==
  imag : Inport
  real : Inport  Port=2
  Concat : xbsIndex_r4/Concat  num_inputs=2  dbl_ovrd=off  block_type=concat
  Reinterpret1 : xbsIndex_r4/Reinterpret  force_arith_type=on  arith_type=Unsigned  force_bin_pt=on  bin_pt=0  block_type=reinterpret
  Reinterpret2 : xbsIndex_r4/Reinterpret  force_arith_type=on  arith_type=Unsigned  force_bin_pt=on  bin_pt=0  block_type=reinterpret
  Slice : xbsIndex_r4/Slice  nbits=1  boolean_output=off  mode=Two Bit Locations  bit1=30  base1=LSB of Input  bit0=15  base0=LSB of Input  dbl_ovrd=off  block_type=slice
  Slice1 : xbsIndex_r4/Slice  nbits=1  boolean_output=off  mode=Two Bit Locations  bit1=30  base1=LSB of Input  bit0=15  base0=LSB of Input  dbl_ovrd=off  block_type=slice
  Out1 : Outport
  wires:
  Slice/1 -> Concat/2
  imag/1 -> Reinterpret2/1
  Concat/1 -> Out1/1
  Slice1/1 -> Concat/1
  real/1 -> Reinterpret1/1
  Reinterpret1/1 -> Slice/1
  Reinterpret2/1 -> Slice1/1

== system syntheses/syntheses/poly_phase_filter/Subsystem2 ==
  ready_in : Inport
  reset_in : Inport  Port=2
  Constant : xbsIndex_r4/Constant  const=N_sub-1  gui_display_data_type=Fixed-point  arith_type=Unsigned  n_bits=nextpow2(N_sub)  bin_pt=0  preci_type=Single  exp_width=8  frac_width=24  explicit_period=off  period=1  equ=P=C  opselect=C  inp2=PCIN>>17  opr=+  inp1=P  carry=CIN  dbl_ovrd=off  block_type=constant
  Constant1 : xbsIndex_r4/Constant  const=1  gui_display_data_type=Boolean  arith_type=Boolean  n_bits=nextpow2(N_sub)  bin_pt=0  preci_type=Single  exp_width=8  frac_width=24  explicit_period=off  period=1  equ=P=C  opselect=C  inp2=PCIN>>17  opr=+  inp1=P  carry=CIN  dbl_ovrd=off  block_type=constant
  Counter : xbsIndex_r4/Counter  cnt_type=Free Running  cnt_to=Inf  operation=Up  start_count=0  cnt_by_val=1  arith_type=Unsigned  n_bits=nextpow2(N_sub)  bin_pt=0  load_pin=off  rst=on  en=on  explicit_period=on  period=1  use_behavioral_HDL=off  implementation=Fabric  dbl_ovrd=off  block_type=counter
  Delay : xbsIndex_r4/Delay  rst=on  infoeditControl=Selection of Reset will increase slice count due to use of real FFs and instead of SRLs  en=on  latency=1  reg_retiming=off  dbl_ovrd=off  block_type=delay
  Inverter : xbsIndex_r4/Inverter  en=off  latency=0  dbl_ovrd=off  block_type=inv
  Relational : xbsIndex_r4/Relational  mode=a=b  op_type=Bool  en=off  latency=0  dbl_ovrd=off  block_type=relational
  valid_out : Outport
  last_out : Outport  Port=2
  data_out : Outport  Port=3
  wires:
  reset_in/1 -> Delay/2, Counter/1
  Counter/1 -> Relational/2, data_out/1
  Constant/1 -> Relational/1
  Relational/1 -> Delay/3, last_out/1
  ready_in/1 -> Counter/2
  Constant1/1 -> Delay/1
  Delay/1 -> Inverter/1
  Inverter/1 -> valid_out/1
